simulink model "TV_2017"  (R2016a)
settings: Solver=FixedStepAuto  StartTime=0.0  StopTime=inf  FixedStep=0.001  RelTol=1e-3
PreLoadFcn:
  | TV_2017_parameters
values from neighbouring files (symbols this model uses):
  battery_voltage = single(530)    [HIL_parameters.m]    (also in HIL_parameters_2018.m; TV_2017_parameters.m; TV_2017_parameters_VD.m)
  car_params = Simulink_Car_params    [HIL_parameters.m]    (also in HIL_parameters_2018.m; TV_2017_parameters.m; TV_2017_parameters_VD.m)
  i_Diff = 16    [HIL_parameters.m]    (also in HIL_parameters_2018.m; TV_2017_parameters.m)
  Kp = 1    [HIL_parameters.m]    (also in HIL_parameters_2018.m; TV_2017_parameters.m; TV_2017_parameters_VD.m)
  motor_data = struct    [HIL_parameters.m]    (also in HIL_parameters_2018.m; TV_2017_parameters.m)
  powerLimitControl = Simulink_el    [HIL_parameters.m]    (also in HIL_parameters_2018.m; TV_2017_parameters.m; TV_2017_parameters_VD.m)
  settings = Simulink_Settings    [HIL_parameters.m]    (also in HIL_parameters_2018.m; TV_2017_parameters.m; TV_2017_parameters_VD.m)
  SpdC_BCC = 0    [HIL_parameters.m]    (also in HIL_parameters_2018.m; TV_2017_parameters.m; TV_2017_parameters_VD.m)
  Speed_Neg_sat = -21    [HIL_parameters.m]    (also in HIL_parameters_2018.m; TV_2017_parameters.m; TV_2017_parameters_VD.m)
  Speed_Pos_sat = 21    [HIL_parameters.m]    (also in HIL_parameters_2018.m; TV_2017_parameters.m; TV_2017_parameters_VD.m)
  SteeringAngleFL = [-23.80 -22.65 -21.50 -20.34 -19.18 -18.03 -16.86 -15.70 -14.53 -13.35 -12.18 -10.99 -9.80 -8.61 -7.40 -6.19 -4.97 -3.75 -2.51 -1.26 0 1.27 2.56 3.85 5.17 6.50 7.84 9.21 10.59 12.00 13.42 14.88 16.36 17.87 19.41 20.99 22.61 24.26 25.97 27.73 29.54]    [CarSetupAnalysis2018.m]    (also in HIL_parameters_2018.m; TV_2017_parameters.m; TV_2017_parameters_VD.m = [-24.129 -22.950 -21.772 -20.593 -19.413 -18.232 -17.050 -15)
  SteeringAngleFR = [-29.54 -27.73 -25.97 -24.26 -22.61 -20.99 -19.41 -17.87 -16.36 -14.88 -13.42 -12.00 -10.59 -9.21 -7.84 -6.50 -5.17 -3.85 -2.56 -1.27 0 1.26 2.51 3.75 4.97 6.19 7.40 8.61 9.80 10.99 12.18 13.35 14.53 15.70 16.86 18.03 19.18 20.34 21.50 22.65 23.80]    [CarSetupAnalysis2018.m]    (also in HIL_parameters_2018.m; TV_2017_parameters.m; TV_2017_parameters_VD.m = [-29.3050 -27.5340 -25.8140 -24.1410 -22.5110 -20.9180 -19.3)
  SteeringWhAngle = [-105 -99.75 -94.5 -89.25 -84 -78.75 -73.5 -68.25 -63 -57.75 -52.5 -47.25 -42 -36.75 -31.5 -26.25 -21.0 -15.75 -10.5 -5.25 0.0 5.25 10.50 15.75 21.00 26.25 31.50 36.75 42.00 47.25 52.50 57.75  63.00 68.25 73.50 78.75 84.00 89.25 94.50 99.75 105.00]    [TV_2017_parameters_VD.m]
  Tn_n = 0    [HIL_parameters.m]    (also in HIL_parameters_2018.m; TV_2017_parameters.m; TV_2017_parameters_VD.m)
  tractionControl = Simulink_tc    [HIL_parameters.m]    (also in HIL_parameters_2018.m; IterativeTractionControlTuning.m; TV_2017_parameters.m; TV_2017_parameters_VD.m)
  yawMomentGenerator = struct    [HIL_parameters.m]    (also in HIL_parameters_2018.m = Simulink_yawRate2; TV_2017_parameters.m = Simulink_yawRate2)
  yawRateControl = Simulink_yawRate    [HIL_parameters.m]    (also in HIL_parameters_2018.m; TV_2017_parameters.m; TV_2017_parameters_VD.m)
undefined symbols (not defined in the file or in its folder): DiscIntNeverNeededParam, magnitude, speedEstimation, TC_Decr_Gas, TC_Derivative, TC_Incr_Gas, TC_On, TC_Relay_Off, TC_Relay_On
libraries: CarMaker4SL x350, simulink_extras x63, simulink x37, dspfdesign x2
(part 13 of 14)

== matlab function TV_2017/CarMaker/Control_System /Output Interface reduce slipratio/MATLAB Function ==
  data: Ti input Bus: Ti_lim; Ti_pos output Bus: Ti_pos; Ti_neg output Bus: Ti_neg; wi_setpoints output Bus: wi_set; settings parameter; car_params parameter
function [Ti_pos, Ti_neg, wi_setpoints] = setPointCalculation(Ti,settings,car_params)
%#codegen

%Conversion factor to calculate RPM limits based on speed limits
%v_to_motor_RPM = single(60*car_params.GR/(2*pi*car_params.r_eff));
not_in_use = settings.RPM_scaling;
max_rpm = settings.max_RPM;
KERS_RPM_setpoint = settings.KERS_motor_RPM_setpoint;
    
%***************** FL ************

if  (Ti.FL <= 0)  
    Ti_pos.FL = int16(0);
    Ti_neg.FL = int16(max(-settings.max_motor_brake_torque/car_params.Mn, Ti.FL/car_params.Mn));
    wi_setpoints.FL = int16(KERS_RPM_setpoint);

elseif Ti.FL > 0
    Ti_pos.FL = int16( Ti.FL/car_params.Mn);
    Ti_neg.FL = int16(0);
    wi_setpoints.FL = int16(max_rpm);  
else
    Ti_pos.FL = int16(0);
    Ti_neg.FL = int16(0);
    wi_setpoints.FL = int16(0); 
end

%***************** FR ************

if  (Ti.FR <= 0)
    Ti_pos.FR = int16(0);
    Ti_neg.FR = int16(max(-settings.max_motor_brake_torque/car_params.Mn, Ti.FR/car_params.Mn));
    wi_setpoints.FR = int16(KERS_RPM_setpoint);

elseif Ti.FR > 0
    Ti_pos.FR = int16( Ti.FR/car_params.Mn);
    Ti_neg.FR = int16(0);
    wi_setpoints.FR = int16(max_rpm);  
else
    Ti_pos.FR = int16(0);
    Ti_neg.FR = int16(0);
    wi_setpoints.FR = int16(0); 
end
%***************** RL ************
if  (Ti.RL <= 0)
    Ti_pos.RL = int16(0);
    Ti_neg.RL = int16(max(-settings.max_motor_brake_torque/car_params.Mn, Ti.RL/car_params.Mn));
    wi_setpoints.RL = int16(KERS_RPM_setpoint);

elseif Ti.RL > 0
    Ti_pos.RL = int16( Ti.RL/car_params.Mn);
    Ti_neg.RL = int16(0);
    wi_setpoints.RL = int16(max_rpm);  
else
    Ti_pos.RL = int16(0);
    Ti_neg.RL = int16(0);
    wi_setpoints.RL = int16(0); 
end

%***************** RR ************
if (Ti.RR <= 0)
    Ti_pos.RR = int16(0);
    Ti_neg.RR = int16(max(-settings.max_motor_brake_torque/car_params.Mn, Ti.RR/car_params.Mn));
    wi_setpoints.RR = int16(KERS_RPM_setpoint);

elseif Ti.RR > 0
    Ti_pos.RR = int16( Ti.RR/car_params.Mn);
    Ti_neg.RR = int16(0);
    wi_setpoints.RR = int16(max_rpm);  
else
    Ti_pos.RR = int16(0);
    Ti_neg.RR = int16(0);
    wi_setpoints.RR = int16(0); 
end



% % The RPM at which KERS is turned off
% RPM_limit_low = settings.KERS_speed_limit_hyst_low*v_to_motor_RPM;
% 
% % The RPM at which KERS is allowed again
% RPM_limit_high = settings.KERS_speed_limit_hyst_high*v_to_motor_RPM;
% 
% 
%    persistent firstIteration;
%    persistent KERS_ALLOWED_FL;
%    persistent KERS_ALLOWED_FR;
%    persistent KERS_ALLOWED_RL;
%    persistent KERS_ALLOWED_RR;
%    
%    
%    % Hysteresis on regenerative input based on RPM to avoid oscillation around 
%    % allowed KERS RPM 
%    if isempty(firstIteration)
%       firstIteration = 2; % Avoid overflow in the register and count 1 again
%       KERS_ALLOWED_FL = uint32(0);
%       KERS_ALLOWED_FR = uint32(0);
%       KERS_ALLOWED_RL = uint32(0);
%       KERS_ALLOWED_RR = uint32(0);
%    else
%        
%        %Hysteris around the minimum RPM Set point
%        if     ( (KERS_ALLOWED_FL == 0) && (states.RPM_FL > RPM_limit_high) )
%            KERS_ALLOWED_FL = uint32(1);
%        elseif ( (KERS_ALLOWED_FL == 1) && (states.RPM_FL < RPM_limit_low) )
%            KERS_ALLOWED_FL = uint32(0);
%        end
%        if     ( (KERS_ALLOWED_FR == 0) && (states.RPM_FR > RPM_limit_high) )
%            KERS_ALLOWED_FR = uint32(1);
%        elseif ( (KERS_ALLOWED_FR == 1) && (states.RPM_FR < RPM_limit_low) )
%            KERS_ALLOWED_FR = uint32(0);
%        end
%        if     ( (KERS_ALLOWED_RL == 0) && (states.RPM_RL > RPM_limit_high) )
%            KERS_ALLOWED_RL = uint32(1);
%        elseif ( (KERS_ALLOWED_RL == 1) && (states.RPM_RL < RPM_limit_low) )
%            KERS_ALLOWED_RL = uint32(0);
%        end
%        if     ( (KERS_ALLOWED_RR == 0) && (states.RPM_RR > RPM_limit_high) )
%            KERS_ALLOWED_RR = uint32(1);
%        elseif ( (KERS_ALLOWED_RR == 1) && (states.RPM_RR < RPM_limit_low) )
%            KERS_ALLOWED_RR = uint32(0);
%        end
%        
%        % Hysteresis around maximum RPM ? 
%        
%    end   
%       
% %***************** FL ************
% 
% if ( (Ti.FL <= 0) && (KERS_ALLOWED_FL == 1) ) 
%     Ti_pos.FL = int16(0);
%     Ti_neg.FL = int16( Ti.FL/car_params.Mn);
%     wi_setpoints.FL = int16(KERS_RPM_setpoint);
% elseif ( (Ti.FL <= 0) && (KERS_ALLOWED_FL == 0) )
%     Ti_pos.FL = int16(0);
%     Ti_neg.FL = int16(0);
%     wi_setpoints.FL = int16(0);
% elseif Ti.FL > 0
%     Ti_pos.FL = int16( Ti.FL/car_params.Mn);
%     Ti_neg.FL = int16(0);
%     wi_setpoints.FL = int16(max_rpm);  
% else
%     Ti_pos.FL = int16(0);
%     Ti_neg.FL = int16(0);
%     wi_setpoints.FL = int16(0); 
% end
% 
% %***************** FR ************
% 
% if ( (Ti.FR <= 0) && (KERS_ALLOWED_FR == 1) ) 
%     Ti_pos.FR = int16(0);
%     Ti_neg.FR = int16( Ti.FR/car_params.Mn);
%     wi_setpoints.FR = int16(KERS_RPM_setpoint);
% elseif ( (Ti.FR <= 0) && (KERS_ALLOWED_FR == 0) )
%     Ti_pos.FR = int16(0);
%     Ti_neg.FR = int16(0);
%     wi_setpoints.FR = int16(0);
% elseif Ti.FR > 0
%     Ti_pos.FR = int16( Ti.FR/car_params.Mn);
%     Ti_neg.FR = int16(0);
%     wi_setpoints.FR = int16(max_rpm);  
% else
%     Ti_pos.FR = int16(0);
%     Ti_neg.FR = int16(0);
%     wi_setpoints.FR = int16(0); 
% end
% %***************** RL ************
% if ( (Ti.RL <= 0) && (KERS_ALLOWED_RL == 1) ) 
%     Ti_pos.RL = int16(0);
%     Ti_neg.RL = int16( Ti.RL/car_params.Mn);
%     wi_setpoints.RL = int16(KERS_RPM_setpoint);
% elseif ( (Ti.RL <= 0) && (KERS_ALLOWED_RL == 0) )
%     Ti_pos.RL = int16(0);
%     Ti_neg.RL = int16(0);
%     wi_setpoints.RL = int16(0);
% elseif Ti.RL > 0
%     Ti_pos.RL = int16( Ti.RL/car_params.Mn);
%     Ti_neg.RL = int16(0);
%     wi_setpoints.RL = int16(max_rpm);  
% else
%     Ti_pos.RL = int16(0);
%     Ti_neg.RL = int16(0);
%     wi_setpoints.RL = int16(0); 
% end
% 
% %***************** RR ************
% if ( (Ti.RR <= 0) && (KERS_ALLOWED_RR == 1) ) 
%     Ti_pos.RR = int16(0);
%     Ti_neg.RR = int16( Ti.RR/car_params.Mn);
%     wi_setpoints.RR = int16(KERS_RPM_setpoint);
% elseif ( (Ti.RR <= 0) && (KERS_ALLOWED_RR == 0) )
%     Ti_pos.RR = int16(0);
%     Ti_neg.RR = int16(0);
%     wi_setpoints.RR = int16(0);
% elseif Ti.RR > 0
%     Ti_pos.RR = int16( Ti.RR/car_params.Mn);
%     Ti_neg.RR = int16(0);
%     wi_setpoints.RR = int16(max_rpm);  
% else
%     Ti_pos.RR = int16(0);
%     Ti_neg.RR = int16(0);
%     wi_setpoints.RR = int16(0); 
% end

end

== matlab function TV_2017/CarMaker/Control_System /MATLAB Function1 ==
  data: pow_red input; constraints_TA input; active_constraints output; Ti_TA input; Ti_SR input; Ti_PL input; maxMotorTorque input; saturated output
function [active_constraints,saturated] = fcn(pow_red,constraints_TA,Ti_TA,Ti_SR,Ti_PL,maxMotorTorque)
%#codegen
mmt = maxMotorTorque;
%the first 4*5 constraints evaluated by TA 
%active_constraints = zeros(1,36,'int8');




i=1;
saturated_constraints = zeros(1,4,'int8');

saturated_constraints(i) = ((Ti_TA.FL*10) >= (mmt.mmt_FL*10 ));i = i+1;
saturated_constraints(i) = ((Ti_TA.FR*10) >= (mmt.mmt_FR*10 ));i = i+1;
saturated_constraints(i) = ((Ti_TA.RL*10) >= (mmt.mmt_RL*10 ));i = i+1;
saturated_constraints(i) = ((Ti_TA.RR*10) >= (mmt.mmt_RR*10 ));i = i+1;
saturated = saturated_constraints;
i=1;
traction_constraints = zeros(1,4,'int8');
traction_constraints(i) = Ti_SR.FL < Ti_TA.FL ; i = i+1;
traction_constraints(i) = Ti_SR.FR < Ti_TA.FR ; i = i+1;
traction_constraints(i) = Ti_SR.RL < Ti_TA.RL ; i = i+1;
traction_constraints(i) = Ti_SR.RR < Ti_TA.RR ; i = i+1;
i=1;
power_constraints = zeros(1,4,'int8');
power_constraints(i) = Ti_PL.FL < Ti_SR.FL ; i = i+1;
power_constraints(i) = Ti_PL.FR < Ti_SR.FR ; i = i+1;
power_constraints(i) = Ti_PL.RL < Ti_SR.RL ; i = i+1;
power_constraints(i) = Ti_PL.RR < Ti_SR.RR ; i = i+1;


%active_constraints = zeros(1,36,'int8');

active_constraints = [  pow_red , saturated_constraints ,  traction_constraints ,  power_constraints ,constraints_TA];

== matlab function TV_2017/CarMaker/Control_System /MATLAB Function2 ==
  data: tot_given output; given input
function tot_given = fcn(given)
%#codegen




tot_given = given.FL + given.FR + given.RL + given.RR;

== matlab function TV_2017/CarMaker/Control_System /Subsystem/Torque allocation QP-/max combined tire torque based on (Fz, SA,mu)  ==
  data: states input; maxMotorTorque output Bus: maxMotorTorque; settings parameter; car_params parameter; tractionControl parameter
function maxMotorTorque = maxTireForce(states,settings,car_params,tractionControl)
%#codegen
% draft scale function     (-x^4-x^2)/3 + -x^6/3  + 1
% calculate max tire force based on F_z and slip angle


% Need to be over a certain velocity for this to work....

v_x = states.V_x;
mu = settings.mu;
GR = car_params.GR;
r = car_params.r_eff;
max_slip = tractionControl.slip_ang_limit;
mmt = settings.max_motor_torque;

F_z_FL = states.Fz_FL;
F_z_FR = states.Fz_FR;
F_z_RL = states.Fz_RL;
F_z_RR = states.Fz_RR;

SA_norm_FL = states.SA_FL/max_slip;
SA_norm_FR = states.SA_FR/max_slip;
SA_norm_RL = states.SA_RL/max_slip;
SA_norm_RR = states.SA_RR/max_slip;

mu_scale_factor_FL = (-SA_norm_FL^4 -SA_norm_FL^2)/3 + -SA_norm_FL^6/3  + 1;
mu_scale_factor_FR = (-SA_norm_FR^4 -SA_norm_FR^2)/3 + -SA_norm_FR^6/3  + 1;
mu_scale_factor_RL = (-SA_norm_RL^4 -SA_norm_RL^2)/3 + -SA_norm_RL^6/3  + 1;
mu_scale_factor_RR = (-SA_norm_RR^4 -SA_norm_RR^2)/3 + -SA_norm_RR^6/3  + 1;

if v_x > 2;
    maxMotorTorque.mmt_FL = F_z_FL * mu_scale_factor_FL *mu * r/ GR ;
    maxMotorTorque.mmt_FR = F_z_FR * mu_scale_factor_FR *mu * r/ GR ;
    maxMotorTorque.mmt_RL = F_z_RL * mu_scale_factor_RL *mu * r/ GR ;
    maxMotorTorque.mmt_RR = F_z_RR * mu_scale_factor_RR *mu * r/ GR ;
else
    maxMotorTorque.mmt_FL = mmt;
    maxMotorTorque.mmt_FR = mmt;
    maxMotorTorque.mmt_RL = mmt;
    maxMotorTorque.mmt_RR = mmt;
end

end

== matlab function TV_2017/CarMaker/Control_System /Subsystem/Torque allocation QP-/max long tire torque based on (FZ , mu) ==
  data: states input; maxMotorTorque output Bus: maxMotorTorque; settings parameter; car_params parameter
function maxMotorTorque = maxTireForce(states,settings, car_params)
%#codegen

% calculate max tire force based on F_z and slip angle
mu = settings.mu;
GR = car_params.GR;
r = car_params.r_eff;

F_z_FL = states.Fz_FL;
F_z_FR = states.Fz_FR;
F_z_RL = states.Fz_RL;
F_z_RR = states.Fz_RR;


maxMotorTorque.mmt_FL = F_z_FL * r * mu / GR ;
maxMotorTorque.mmt_FR = F_z_FR * r * mu / GR ;
maxMotorTorque.mmt_RL = F_z_RL * r * mu / GR ;
maxMotorTorque.mmt_RR = F_z_RR * r * mu / GR ;

== matlab function TV_2017/CarMaker/Control_System /Subsystem/Torque allocation QP-/max torque  ==
  data: mu_lim input; SA_lim input; maxMotorTorque output Bus: maxMotorTorque; active_constraints output; inv_temp_lim input; mot_temp_lim input; settings parameter
function [maxMotorTorque, active_constraints] = maxTireForce(mu_lim,SA_lim,inv_temp_lim,mot_temp_lim, settings)
%#codegen
active_constraints = zeros(1,(6*4),'int8');

default_max_torque = settings.max_motor_torque;
default_min_torque = settings.max_motor_brake_torque;
%calc_pow_lim.mmt_FL,
FL_max = max(0,min([inv_temp_lim.mmt_FL,mot_temp_lim.mmt_FL,mu_lim.mmt_FL,SA_lim.mmt_FL,default_max_torque]));
FR_max = max(0,min([inv_temp_lim.mmt_FR,mot_temp_lim.mmt_FR,mu_lim.mmt_FR,SA_lim.mmt_FR,default_max_torque]));
RL_max = max(0,min([inv_temp_lim.mmt_RL,mot_temp_lim.mmt_RL,mu_lim.mmt_RL,SA_lim.mmt_RL,default_max_torque]));
RR_max = max(0,min([inv_temp_lim.mmt_RR,mot_temp_lim.mmt_RR,mu_lim.mmt_RR,SA_lim.mmt_RR,default_max_torque]));

maxMotorTorque.mmt_FL = FL_max;
maxMotorTorque.mmt_FR = FR_max;
maxMotorTorque.mmt_RL = RL_max;
maxMotorTorque.mmt_RR = RR_max;

i = 1;
% active_constraints(i) = isequal(calc_pow_lim.mmt_FL,FL_max); i = i+1;
% active_constraints(i) = isequal(calc_pow_lim.mmt_FR,FR_max); i = i+1;
% active_constraints(i) = isequal(calc_pow_lim.mmt_RL,RL_max); i = i+1;
% active_constraints(i) = isequal(calc_pow_lim.mmt_RR,RR_max); i = i+1;
default_lim_FL = isequal(default_max_torque,FL_max);   %returns 1 if default max torque is the active limit
default_lim_FR = isequal(default_max_torque,FR_max);
default_lim_RL = isequal(default_max_torque,RL_max);
default_lim_RR = isequal(default_max_torque,RR_max);

active_constraints(i) = default_lim_FL;  i = i+1;
active_constraints(i) = default_lim_FR;  i = i+1;
active_constraints(i) = default_lim_RL;  i = i+1;
active_constraints(i) = default_lim_RR;  i = i+1;
% Available power
active_constraints(i) = 0;%isequal(calc_pow_lim.mmt_FL,FL_max) *(1- default_lim_FL) ; i = i+1;
active_constraints(i) = 0;%isequal(calc_pow_lim.mmt_FR,FR_max) *(1- default_lim_FR) ; i = i+1;
active_constraints(i) = 0;%isequal(calc_pow_lim.mmt_RL,RL_max) *(1- default_lim_RL) ; i = i+1;
active_constraints(i) = 0;%isequal(calc_pow_lim.mmt_RR,RR_max) *(1- default_lim_RR) ; i = i+1;
% Inverter temperature
active_constraints(i) = isequal(inv_temp_lim.mmt_FL,FL_max) *(1- default_lim_FL) ;  i = i+1;
active_constraints(i) = isequal(inv_temp_lim.mmt_FR,FR_max) *(1- default_lim_FR) ;  i = i+1;
active_constraints(i) = isequal(inv_temp_lim.mmt_RL,RL_max) *(1- default_lim_RL) ;  i = i+1;
active_constraints(i) = isequal(inv_temp_lim.mmt_RR,RR_max) *(1- default_lim_RR) ;  i = i+1;
%Motor temperature
active_constraints(i) = isequal(mot_temp_lim.mmt_FL,FL_max) *(1- default_lim_FL) ;  i = i+1;
active_constraints(i) = isequal(mot_temp_lim.mmt_FR,FR_max) *(1- default_lim_FR) ;  i = i+1;
active_constraints(i) = isequal(mot_temp_lim.mmt_RL,RL_max) *(1- default_lim_RL) ;  i = i+1;
active_constraints(i) = isequal(mot_temp_lim.mmt_RR,RR_max) *(1- default_lim_RR) ;  i = i+1;
% Friction square
active_constraints(i) = isequal(mu_lim.mmt_FL,FL_max) *(1- default_lim_FL) ;  i = i+1;
active_constraints(i) = isequal(mu_lim.mmt_FR,FR_max) *(1- default_lim_FR) ;  i = i+1;
active_constraints(i) = isequal(mu_lim.mmt_RL,RL_max) *(1- default_lim_RL) ;  i = i+1;
active_constraints(i) = isequal(mu_lim.mmt_RR,RR_max) *(1- default_lim_RR) ;  i = i+1;
% friction ellipse
active_constraints(i) = isequal(SA_lim.mmt_FL,FL_max) *(1- default_lim_FL) ;  i = i+1;
active_constraints(i) = isequal(SA_lim.mmt_FR,FR_max) *(1- default_lim_FR) ;  i = i+1;
active_constraints(i) = isequal(SA_lim.mmt_RL,RL_max) *(1- default_lim_RL) ;  i = i+1;
active_constraints(i) = isequal(SA_lim.mmt_RR,RR_max) *(1- default_lim_RR) ;  i = i+1;


%active_constraints(i) = i;  i = i+1;
 

%active_constraints

== matlab function TV_2017/CarMaker/Control_System /Subsystem/Torque allocation QP-/maxMotorTorque and kers based on available power ==
  data: states input; maxMotorTorque output Bus: maxMotorTorque; settings parameter; kers_allowed output
function [maxMotorTorque,kers_allowed] = MaxMotorTorque_Power(states,settings)
%#codegen

% DC Voltage                             / states
% Max allowable current draw in total    /settings
% Load distribution                      /states






if states.V_x<=settings.KERS_speed_limit_hyst_low
    kers_allowed = single(0);
elseif states.V_x>=settings.KERS_speed_limit_hyst_high
    kers_allowed = single(1);
else
    kers_allowed = single(0);
end

Fzi = [max(1,states.Fz_FL) max(1,states.Fz_FR) max(1,states.Fz_RL) max(1,states.Fz_RR)]';

switch settings.TV_Method
    case 1 % No negative torque
        alfa_r =  (Fzi(3) + Fzi(4)) / (Fzi(1) + Fzi(2) + Fzi(3) + Fzi(4));
    case 2 % with negative torque
        alfa_r =  (Fzi(3) + Fzi(4)) / (Fzi(1) + Fzi(2) + Fzi(3) + Fzi(4));
    case 3 % static 25 %
        alfa_r = single(0.5);
    case 4 % with negative torque, no Fz
        alfa_r = single(0.5);
    otherwise
        alfa_r = single(0.5);
end

RPM_to_angular = single(2*pi/60);
omega_FL = states.RPM_FL*RPM_to_angular;
omega_FR = states.RPM_FR*RPM_to_angular;
omega_RL = states.RPM_RL*RPM_to_angular;
omega_RR = states.RPM_RR*RPM_to_angular;

mmt = settings.max_motor_torque;
available_power = states.DC_voltage*settings.max_battery_discharge;

max_torque_front = min(mmt, (available_power*(1-alfa_r))/ (2 * max( max(1,omega_FL), max(1,omega_FR))) );
max_torque_rear = min(mmt, (available_power*alfa_r)     / (2 * max( max(1,omega_RL), max(1,omega_RR))) );
                      
maxMotorTorque.mmt_FL = max_torque_front;
maxMotorTorque.mmt_FR = max_torque_front;
maxMotorTorque.mmt_RL = max_torque_rear;
maxMotorTorque.mmt_RR = max_torque_rear;

== matlab function TV_2017/CarMaker/Control_System /Subsystem/2016 adapted/Inverter temperature limiter ==
  data: states input; maxMotorTorque output Bus: maxMotorTorque; settings parameter; car_params parameter
function maxMotorTorque = maxMotorTorque_InvTemp(states,settings, car_params)
%#codegen

% The inverters limits output torque based on internal temperature
mmt                 =  single(settings.max_motor_torque);
upper_max_temp      =  single(car_params.AMK_inverter_upper_max_temp);
cutoff_temp         =  single(car_params.AMK_inverter_cutoff_temp);

torque = [mmt, mmt, single(0)]; %breakpoints for lookup function
temp = [single(0), upper_max_temp, cutoff_temp];

inv_FL_temp = single(states.AMK_inverter_temp_FL);
inv_FR_temp = single(states.AMK_inverter_temp_FR);
inv_RL_temp = single(states.AMK_inverter_temp_RL);
inv_RR_temp = single(states.AMK_inverter_temp_RR);

%  y = interp1(xdata,ydata,x)
maxMotorTorque.mmt_FL = interp1(  temp , torque,  inv_FL_temp  );
maxMotorTorque.mmt_FR = interp1(  temp , torque,  inv_FR_temp  );
maxMotorTorque.mmt_RL = interp1(  temp , torque,  inv_RL_temp  );
maxMotorTorque.mmt_RR = interp1(  temp , torque,  inv_RR_temp  );

== matlab function TV_2017/CarMaker/Control_System /Subsystem/2016 adapted/Motor temperature limiter ==
  data: states input; maxMotorTorque output Bus: maxMotorTorque; settings parameter; car_params parameter
function maxMotorTorque = maxMotorTorque_MotorTemp(states,settings, car_params)
%#codegen

% The inverters limits output torque based on internal temperature
mmt = single(settings.max_motor_torque);
upper_max_temp = single(car_params.AMK_motor_upper_max_temp);
cutoff_temp    = single(car_params.AMK_motor_cutoff_temp);
torque = [mmt mmt 0]; %breakpoints for lookup function
temp = [0 upper_max_temp cutoff_temp];


mot_FL_temp = single(states.AMK_inverter_temp_FL);
mot_FR_temp = single(states.AMK_inverter_temp_RL);
mot_RL_temp = single(states.AMK_inverter_temp_RL);
mot_RR_temp = single(states.AMK_inverter_temp_RR);

%  y = interp1(xdata,ydata,x)
maxMotorTorque.mmt_FL = interp1(temp,torque,  mot_FL_temp  );
maxMotorTorque.mmt_FR = interp1(temp,torque,  mot_FR_temp  );
maxMotorTorque.mmt_RL = interp1(temp,torque,  mot_RL_temp  );
maxMotorTorque.mmt_RR = interp1(temp,torque,  mot_RR_temp  );

== matlab function TV_2017/CarMaker/Control_System /Subsystem/2016 adapted/max combined tire torque based on (Fz, SA,mu)  ==
  data: states input; maxMotorTorque output Bus: maxMotorTorque; settings parameter; car_params parameter; tractionControl parameter
function maxMotorTorque = maxTireForce(states,settings,car_params,tractionControl)
%#codegen
% draft scale function     (-x^4-x^2)/3 + -x^6/3  + 1
% calculate max tire force based on F_z and slip angle
mu = settings.mu;
GR = car_params.GR;
r = car_params.r_eff;
max_slip = tractionControl.slip_ang_limit;

F_z_FL = states.Fz_FL;
F_z_FR = states.Fz_FR;
F_z_RL = states.Fz_RL;
F_z_RR = states.Fz_RR;

SA_norm_FL = states.SA_FL/max_slip;
SA_norm_FR = states.SA_FR/max_slip;
SA_norm_RL = states.SA_RL/max_slip;
SA_norm_RR = states.SA_RR/max_slip;

mu_scale_factor_FL = (-SA_norm_FL^4 -SA_norm_FL^2)/3 + -SA_norm_FL^6/3  + 1;
mu_scale_factor_FR = (-SA_norm_FR^4 -SA_norm_FR^2)/3 + -SA_norm_FR^6/3  + 1;
mu_scale_factor_RL = (-SA_norm_RL^4 -SA_norm_RL^2)/3 + -SA_norm_RL^6/3  + 1;
mu_scale_factor_RR = (-SA_norm_RR^4 -SA_norm_RR^2)/3 + -SA_norm_RR^6/3  + 1;

maxMotorTorque.mmt_FL = F_z_FL * mu_scale_factor_FL *mu * r/ GR ;
maxMotorTorque.mmt_FR = F_z_FR * mu_scale_factor_FR *mu * r/ GR ;
maxMotorTorque.mmt_RL = F_z_RL * mu_scale_factor_RL *mu * r/ GR ;
maxMotorTorque.mmt_RR = F_z_RR * mu_scale_factor_RR *mu * r/ GR ;

== matlab function TV_2017/CarMaker/Control_System /Subsystem/2016 adapted/max long tire torque based on (FZ , mu) ==
  data: states input; maxMotorTorque output Bus: maxMotorTorque; settings parameter; car_params parameter
function maxMotorTorque = maxTireForce(states,settings, car_params)
%#codegen

% calculate max tire force based on F_z and slip angle
mu = settings.mu;
GR = car_params.GR;
r = car_params.r_eff;

F_z_FL = states.Fz_FL;
F_z_FR = states.Fz_FR;
F_z_RL = states.Fz_RL;
F_z_RR = states.Fz_RR;


maxMotorTorque.mmt_FL = F_z_FL * r * mu / GR ;
maxMotorTorque.mmt_FR = F_z_FR * r * mu / GR ;
maxMotorTorque.mmt_RL = F_z_RL * r * mu / GR ;
maxMotorTorque.mmt_RR = F_z_RR * r * mu / GR ;

== matlab function TV_2017/CarMaker/Control_System /Subsystem/2016 adapted/max torque  ==
  data: maxMotorTorque output Bus: maxMotorTorque; calc_pow_lim input; active_constraints output; inv_temp_lim input; mot_temp_lim input; mu_lim input; SA_lim input; settings parameter
function [maxMotorTorque, active_constraints] = maxTireForce(calc_pow_lim,inv_temp_lim,mot_temp_lim,mu_lim,SA_lim, settings)
%#codegen
active_constraints = zeros(1,(6*4),'int8');

default_max_torque = settings.max_motor_torque;
default_min_torque = settings.max_motor_brake_torque;

FL_max = min([calc_pow_lim.mmt_FL,inv_temp_lim.mmt_FL,mot_temp_lim.mmt_FL,mu_lim.mmt_FL,SA_lim.mmt_FL,default_max_torque]);
FR_max = min([calc_pow_lim.mmt_FR,inv_temp_lim.mmt_FR,mot_temp_lim.mmt_FR,mu_lim.mmt_FR,SA_lim.mmt_FR,default_max_torque]);
RL_max = min([calc_pow_lim.mmt_RL,inv_temp_lim.mmt_RL,mot_temp_lim.mmt_RL,mu_lim.mmt_RL,SA_lim.mmt_RL,default_max_torque]);
RR_max = min([calc_pow_lim.mmt_RR,inv_temp_lim.mmt_RR,mot_temp_lim.mmt_RR,mu_lim.mmt_RR,SA_lim.mmt_RR,default_max_torque]);

maxMotorTorque.mmt_FL = FL_max;
maxMotorTorque.mmt_FR = FR_max;
maxMotorTorque.mmt_RL = RL_max;
maxMotorTorque.mmt_RR = RR_max;


% active_constraints(i) = isequal(calc_pow_lim.mmt_FL,FL_max); i = i+1;
% active_constraints(i) = isequal(calc_pow_lim.mmt_FR,FR_max); i = i+1;
% active_constraints(i) = isequal(calc_pow_lim.mmt_RL,RL_max); i = i+1;
% active_constraints(i) = isequal(calc_pow_lim.mmt_RR,RR_max); i = i+1;
default_lim_FL = isequal(default_max_torque,FL_max);   %returns 1 if default max torque is the active limit
default_lim_FR = isequal(default_max_torque,FR_max);
default_lim_RL = isequal(default_max_torque,RL_max);
default_lim_RR = isequal(default_max_torque,RR_max);

i = 1;
%default limit max motor torque
active_constraints(i) = default_lim_FL;  i = i+1;
active_constraints(i) = default_lim_FR;  i = i+1;
active_constraints(i) = default_lim_RL;  i = i+1;
active_constraints(i) = default_lim_RR;  i = i+1;
% Available power
active_constraints(i) = isequal(calc_pow_lim.mmt_FL,FL_max) *(1- default_lim_FL) ; i = i+1;
active_constraints(i) = isequal(calc_pow_lim.mmt_FR,FR_max) *(1- default_lim_FR) ; i = i+1;
active_constraints(i) = isequal(calc_pow_lim.mmt_RL,RL_max) *(1- default_lim_RL) ; i = i+1;
active_constraints(i) = isequal(calc_pow_lim.mmt_RR,RR_max) *(1- default_lim_RR) ; i = i+1;
% Inverter temperature
active_constraints(i) = isequal(inv_temp_lim.mmt_FL,FL_max) *(1- default_lim_FL) ;  i = i+1;
active_constraints(i) = isequal(inv_temp_lim.mmt_FR,FR_max) *(1- default_lim_FR) ;  i = i+1;
active_constraints(i) = isequal(inv_temp_lim.mmt_RL,RL_max) *(1- default_lim_RL) ;  i = i+1;
active_constraints(i) = isequal(inv_temp_lim.mmt_RR,RR_max) *(1- default_lim_RR) ;  i = i+1;
%Motor temperature
active_constraints(i) = isequal(mot_temp_lim.mmt_FL,FL_max) *(1- default_lim_FL) ;  i = i+1;
active_constraints(i) = isequal(mot_temp_lim.mmt_FR,FR_max) *(1- default_lim_FR) ;  i = i+1;
active_constraints(i) = isequal(mot_temp_lim.mmt_RL,RL_max) *(1- default_lim_RL) ;  i = i+1;
active_constraints(i) = isequal(mot_temp_lim.mmt_RR,RR_max) *(1- default_lim_RR) ;  i = i+1;
% Friction square
active_constraints(i) = isequal(mu_lim.mmt_FL,FL_max) *(1- default_lim_FL) ;  i = i+1;
active_constraints(i) = isequal(mu_lim.mmt_FR,FR_max) *(1- default_lim_FR) ;  i = i+1;
active_constraints(i) = isequal(mu_lim.mmt_RL,RL_max) *(1- default_lim_RL) ;  i = i+1;
active_constraints(i) = isequal(mu_lim.mmt_RR,RR_max) *(1- default_lim_RR) ;  i = i+1;
% friction ellipse
active_constraints(i) = isequal(SA_lim.mmt_FL,FL_max) *(1- default_lim_FL) ;  i = i+1;
active_constraints(i) = isequal(SA_lim.mmt_FR,FR_max) *(1- default_lim_FR) ;  i = i+1;
active_constraints(i) = isequal(SA_lim.mmt_RL,RL_max) *(1- default_lim_RL) ;  i = i+1;
active_constraints(i) = isequal(SA_lim.mmt_RR,RR_max) *(1- default_lim_RR) ;  i = i+1;


%active_constraints(i) = i;  i = i+1;
 

active_constraints;

== matlab function TV_2017/CarMaker/Control_System /Subsystem/2016 adapted/maxMotorTorque and kers based on available power ==
  data: states input; maxMotorTorque output Bus: maxMotorTorque; settings parameter; kers_allowed output
function [maxMotorTorque,kers_allowed] = MaxMotorTorque_Power(states,settings)
%#codegen

% DC Voltage                             / states
% Max allowable current draw in total    /settings
% Load distribution                      /states






if states.V_x<=settings.KERS_speed_limit_hyst_low
    kers_allowed = single(0);
elseif states.V_x>=settings.KERS_speed_limit_hyst_high
    kers_allowed = single(1);
else
    kers_allowed = single(0);
end

Fzi = [max(1,states.Fz_FL) max(1,states.Fz_FR) max(1,states.Fz_RL) max(1,states.Fz_RR)]';

switch settings.TV_Method
    case 1 % No negative torque
        alfa_r =  (Fzi(3) + Fzi(4)) / (Fzi(1) + Fzi(2) + Fzi(3) + Fzi(4));
    case 2 % with negative torque
        alfa_r =  (Fzi(3) + Fzi(4)) / (Fzi(1) + Fzi(2) + Fzi(3) + Fzi(4));
    case 3 % static 25 %
        alfa_r = single(0.5);
    case 4 % with negative torque, no Fz
        alfa_r = single(0.5);
    otherwise
        alfa_r = single(0.5);
end

RPM_to_angular = single(2*pi/60);
omega_FL = states.RPM_FL*RPM_to_angular;
omega_FR = states.RPM_FR*RPM_to_angular;
omega_RL = states.RPM_RL*RPM_to_angular;
omega_RR = states.RPM_RR*RPM_to_angular;

mmt = settings.max_motor_torque;
available_power = states.DC_voltage*settings.max_battery_discharge;

max_torque_front = min(mmt, (available_power*(1-alfa_r))/ (2 * max( max(1,omega_FL), max(1,omega_FR))) );
max_torque_rear = min(mmt, (available_power*alfa_r)     / (2 * max( max(1,omega_RL), max(1,omega_RR))) );
                      
maxMotorTorque.mmt_FL = max_torque_front;
maxMotorTorque.mmt_FR = max_torque_front;
maxMotorTorque.mmt_RL = max_torque_rear;
maxMotorTorque.mmt_RR = max_torque_rear;

== matlab function TV_2017/CarMaker/Control_System /Subsystem/Torque allocation QP-1/Inverter temperature limiter ==
  data: states input; maxMotorTorque output Bus: maxMotorTorque; settings parameter; car_params parameter
function maxMotorTorque = maxMotorTorque_InvTemp(states,settings, car_params)
%#codegen
inv_FL_temp =int16(20);
inv_FR_temp =20;
inv_RL_temp =20;
inv_RR_temp =20;


% The inverters limits output torque based on internal temperature
mmt                 =  single(settings.max_motor_torque);
upper_max_temp      =  single(car_params.AMK_inverter_upper_max_temp);
cutoff_temp         =  single(car_params.AMK_inverter_cutoff_temp);

torque = [mmt, mmt, single(0)]; %breakpoints for lookup function
temp = [single(0), upper_max_temp, cutoff_temp];

inv_FL_temp = single(states.AMK_inverter_temp_FL);
inv_FR_temp = single(states.AMK_inverter_temp_FR);
inv_RL_temp = single(states.AMK_inverter_temp_RL);
inv_RR_temp = single(states.AMK_inverter_temp_RR);

%  y = interp1(xdata,ydata,x)
maxMotorTorque.mmt_FL = interp1(  temp , torque,  inv_FL_temp  );
maxMotorTorque.mmt_FR = interp1(  temp , torque,  inv_FR_temp  );
maxMotorTorque.mmt_RL = interp1(  temp , torque,  inv_RL_temp  );
maxMotorTorque.mmt_RR = interp1(  temp , torque,  inv_RR_temp  );

== matlab function TV_2017/CarMaker/Control_System /Subsystem/Torque allocation QP-1/Motor temperature limiter ==
  data: states input; maxMotorTorque output Bus: maxMotorTorque; settings parameter; car_params parameter
function maxMotorTorque = maxMotorTorque_MotorTemp(states,settings, car_params)
%#codegen

% The inverters limits output torque based on internal temperature
mmt = single(settings.max_motor_torque);
upper_max_temp = single(car_params.AMK_motor_upper_max_temp);
cutoff_temp    = single(car_params.AMK_motor_cutoff_temp);
torque = [mmt mmt 0]; %breakpoints for lookup function
temp = [0 upper_max_temp cutoff_temp];


mot_FL_temp = single(states.AMK_inverter_temp_FL);
mot_FR_temp = single(states.AMK_inverter_temp_RL);
mot_RL_temp = single(states.AMK_inverter_temp_RL);
mot_RR_temp = single(states.AMK_inverter_temp_RR);

%  y = interp1(xdata,ydata,x)
maxMotorTorque.mmt_FL = interp1(temp,torque,  mot_FL_temp  );
maxMotorTorque.mmt_FR = interp1(temp,torque,  mot_FR_temp  );
maxMotorTorque.mmt_RL = interp1(temp,torque,  mot_RL_temp  );
maxMotorTorque.mmt_RR = interp1(temp,torque,  mot_RR_temp  );

== matlab function TV_2017/CarMaker/Estimations/Subsystem/Slip_Detection/Slip Detection ==
  data: SR input; sensors input; slip_prev input Bus: SR; slip output Bus: SR; tractionControl parameter; car_params parameter
function slip = slipDetection(SR , sensors , slip_prev , tractionControl , car_params)
%#codegen
slip_rate_pos_lim = single(tractionControl.slip_rate_pos_lim); % dette må legges inn i carParameters
slip_rate_neg_lim = single(tractionControl.slip_rate_neg_lim);
omega_der_slip_lim = single(tractionControl.omega_der_slip_lim);
omega_der_lock_lim = single(tractionControl.omega_der_lock_lim);

GR = car_params.GR;
% Convert RPM Derivative to angular acceleration in radians per second. 
c = single(2*pi/(GR*60));
ang_acc_FL = c*sensors.RPM_der_FL;
ang_acc_FR = c*sensors.RPM_der_FR;
ang_acc_RL = c*sensors.RPM_der_RL;
ang_acc_RR = c*sensors.RPM_der_RR;

% Slip rate, thypical values between -1 and 1;
SR_FL = SR.FL;
SR_FR = SR.FR;
SR_RL = SR.RL;
SR_RR = SR.RR;

slip_prev_FL = slip_prev.FL;
slip_prev_FR = slip_prev.FR;
slip_prev_RL = slip_prev.RL;
slip_prev_RR = slip_prev.RR;

% detection criteria for slip. Check documentation on drive/confluence from
% testing this on analyze data.
if    ((ang_acc_FL > omega_der_slip_lim && SR_FL > 0)  || (SR_FL > slip_rate_pos_lim && slip_prev_FL ==  1))
   slip_FL = single(1);
elseif((ang_acc_FL < omega_der_lock_lim && SR_FL < 0)  || (SR_FL < slip_rate_neg_lim && slip_prev_FL == -1))
   slip_FL = single(-1);
else
   slip_FL = single(0);
end

if    ( (ang_acc_FR > omega_der_slip_lim && SR_FR > 0 ) || (SR_FR > slip_rate_pos_lim && slip_prev_FR ==  1))
   slip_FR = single(1);
elseif( (ang_acc_FR < omega_der_lock_lim && SR_FR < 0 ) || (SR_FR < slip_rate_neg_lim && slip_prev_FR == -1))
   slip_FR = single(-1);
else
   slip_FR = single(0);
end

if    ( (ang_acc_RL > omega_der_slip_lim && SR_RL > 0)  || (SR_RL > slip_rate_pos_lim && slip_prev_RL ==  1) )
   slip_RL = single(1);
elseif( (ang_acc_RL < omega_der_lock_lim && SR_RL < 0)  || (SR_RL < slip_rate_neg_lim && slip_prev_RL == -1) )
   slip_RL = single(-1);
else
   slip_RL = single(0);
end

if    ( (ang_acc_RR > omega_der_slip_lim && SR_RR > 0)  || (SR_RR > slip_rate_pos_lim && slip_prev_RR ==  1) )
   slip_RR = single(1);
elseif( (ang_acc_RR < omega_der_lock_lim && SR_RR < 0)  || (SR_RR < slip_rate_neg_lim && slip_prev_RR == -1) )
   slip_RR = single(-1);
else
   slip_RR = single(0);
end

slip.FL = slip_FL;
slip.FR = slip_FR;
slip.RL = slip_RL;
slip.RR = slip_RR;
end

== matlab function TV_2017/CarMaker/Control_System /TA 2017/Slip handling (Traction Control) /Scaling factors from slip detection ==
  data: states input; prev_duration input Bus: SlipDuration; prev_slip input Bus: SlipStorage; slipScalingFactor output Bus: SlipStorage; duration output Bus: SlipDuration; tractionControl parameter; slip output Bus: SlipStorage
function [slipScalingFactor ,duration , slip] = slipScalingFactors(states, prev_duration, prev_slip, tractionControl)
%#codegen
% Making s scaling factor for the estimated capacity  on the wheels when
% slip is detected. 
% Starts by scaling down by a constant factor between 0 and 1, and then
% letting it grow smoothly up to 1 again. 
% Uses different start value for slip/lock, but has the same growth rate. 
% Riset time is given as the time it takes to rise from 0 to 1. (so with a
% scaling factor of 0.5, it wil use half of the risetime to get back to 1.

persistent scale_FL;
persistent scale_FR;
persistent scale_RL;
persistent scale_RR;
persistent dur_FL;
persistent dur_FR;
persistent dur_RL;
persistent dur_RR;
persistent firstIteration;

enable = tractionControl.enable2;
V_x=  states.V_x;
riseTime = max(1,tractionControl.riseTime); 
growthFactor = single(1/riseTime);
startValueSlip = tractionControl.startValueSlip;
startValueLock = tractionControl.startValueLock;
startSlip = single(startValueSlip/growthFactor);
startLock = single(startValueLock/growthFactor);


if isempty(firstIteration)
    firstIteration = 2; % Initializing
    dur_FL = single(riseTime);
    dur_FR = single(riseTime);
    dur_RL = single(riseTime);
    dur_RR = single(riseTime);
    scale_FL = single(1);
    scale_FR = single(1);
    scale_RL = single(1);
    scale_RR = single(1);
else
    dur_FL  = single(prev_duration.FL); 
    dur_FR  = single(prev_duration.FR); 
    dur_RL  = single(prev_duration.RL); 
    dur_RR  = single(prev_duration.RR);
end



slip_FL = states.slip_FL;
slip_FR = states.slip_FR;
slip_RL = states.slip_RL;
slip_RR = states.slip_RR;
 
if(enable && (V_x <= 30))
    %Wheel lock (KERS)
    if (slip_FL == -1 && prev_slip.FL == 0)
        dur_FL = single(startLock);
    end
    if (slip_FR == -1 && prev_slip.FR == 0)
        dur_FR = single(startLock);
    end
    if (slip_RL == -1 && prev_slip.RL == 0)
        dur_RL = single(startLock);
    end
    if (slip_RR == -1 && prev_slip.RR == 0)
        dur_RR = single(startLock);
    end

    %Wheel slip
    if (slip_FL == 1 && prev_slip.FL == 0)
        dur_FL = single(startSlip);
    end
    if (slip_FR == 1 && prev_slip.FR == 0)
        dur_FR = single(startSlip);
    end
    if (slip_RL == 1 && prev_slip.RL == 0)
        dur_RL = single(startSlip);
    end
    if (slip_RR == 1 && prev_slip.RR == 0)
        dur_RR = single(startSlip);
    end

    % makes the scaling rise back to 1
    if(dur_FL <= riseTime)
        scale_FL = growthFactor * dur_FL;
        dur_FL = dur_FL +1;
    end
    if(dur_FR <= riseTime)
        scale_FR = growthFactor * dur_FR;
        dur_FR = dur_FR +1;
    end
    if(dur_RL <= riseTime)
        scale_RL = growthFactor * dur_RL;
        dur_RL = dur_RL +1;
    end
    if(dur_RR <= riseTime)
        scale_RR = growthFactor * dur_RR;
        dur_RR = dur_RR +1;
    end

    %sets the scaling factor (the actual output of this function)
    slipScalingFactor.FL = single(1);
    slipScalingFactor.FR = single(1);
    slipScalingFactor.RL = single(1);
    slipScalingFactor.RR = single(1);
else
    slipScalingFactor.FL = single(1); %no scaling
    slipScalingFactor.FR = single(1);
    slipScalingFactor.RL = single(1);
    slipScalingFactor.RR = single(1);
end

%set duration for memoryloop.
duration.FL = dur_FL;
duration.FR = dur_FR;
duration.RL = dur_RL;
duration.RR = dur_RR;
%set slip state for memoryloop
slip.FL = slip_FL;
slip.FR = slip_FR;
slip.RL = slip_RL;
slip.RR = slip_RR;
end
